simulink model "test_block"  (R2022b)
settings: Solver=VariableStepAuto  StartTime=0.0  StopTime=10.0  RelTol=1e-3
settings Model: Creator=phatdo  LastModifiedBy=phatdo

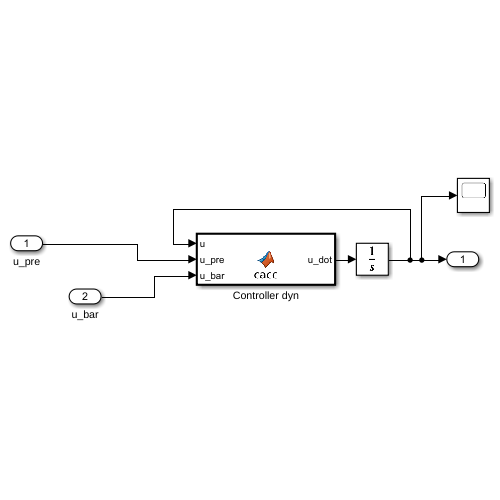
[thumbnail: Simulink's stored preview of the top-level diagram]
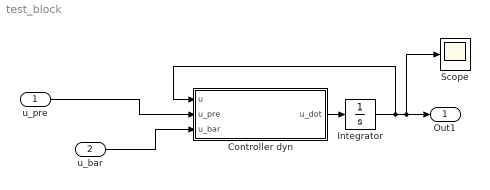
== system test_block ==
  u_pre : Inport
  u_bar : Inport  Port=2
  Controller dyn : MATLAB Function  TreatAsAtomicUnit=on
  Integrator : Integrator  InitialCondition=5
  Scope : Scope
  Out1 : Outport
  wires:
  Controller dyn/1(u_dot) -> Integrator/1
  u_bar/1 -> Controller dyn/3(u_bar)
  Integrator/1 -> Controller dyn/1(u), Scope/1, Out1/1
  u_pre/1 -> Controller dyn/2(u_pre)

== matlab function test_block/Controller dyn ==
  data: u input; u_dot output; u_pre input; u_bar input
function u_dot = cacc(u, u_pre, u_bar)

h = 1; % second

u_dot = -1/h * u;

end
